simulink model "padego"  (Simulink 7.9)
settings: Solver=ode4  StartTime=0.0  StopTime=10.0  FixedStep=0.01  RelTol=1e-3
values from neighbouring files (symbols this model uses):
  K = 1    [scr.m]
  T = 1    [scr.m]
  theta = X0(1)    [pade_err.m]    (also in scr.m = 0.9641)
settings Model: Creator=student  LastModifiedBy=student

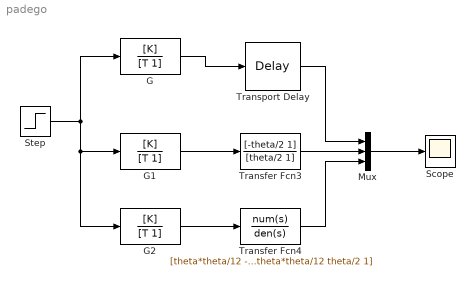
== system padego ==
  G : TransferFcn  Numerator=[K]  Denominator=[T 1]
  G1 : TransferFcn  Numerator=[K]  Denominator=[T 1]
  G2 : TransferFcn  Numerator=[K]  Denominator=[T 1]
  Mux : Mux  Inputs=3
  Scope : Scope
  Step : Step  Time=0  SampleTime=0
  Transfer Fcn3 : TransferFcn  Numerator=[-theta/2 1]  Denominator=[theta/2 1]
  Transfer Fcn4 : TransferFcn  Numerator=[theta*theta/12 -theta/2 1]  Denominator=[theta*theta/12 theta/2 1]
  Transport Delay : TransportDelay  DelayTime=theta
  wires:
  Step/1 -> G/1, G1/1, G2/1
  G/1 -> Transport Delay/1
  G1/1 -> Transfer Fcn3/1
  G2/1 -> Transfer Fcn4/1
  Transport Delay/1 -> Mux/1
  Transfer Fcn3/1 -> Mux/2
  Transfer Fcn4/1 -> Mux/3
  Mux/1 -> Scope/1
